simulink model "c_spacecraft_control_sensors_noise_removal"  (R2022a)
settings: Solver=ode45  StartTime=0.0  StopTime=30  RelTol=1e-3
undefined symbols (not defined in the file): Continuous, Time
libraries: slpidlib x3, aerolibnav x1, ctrlSharedLib x1, simulink x1, robotcorelib x1
settings Model: Creator=HP  LastModifiedBy=HP

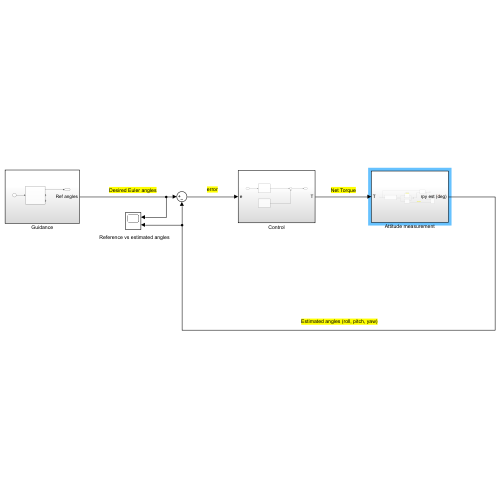
[thumbnail: Simulink's stored preview of the top-level diagram]
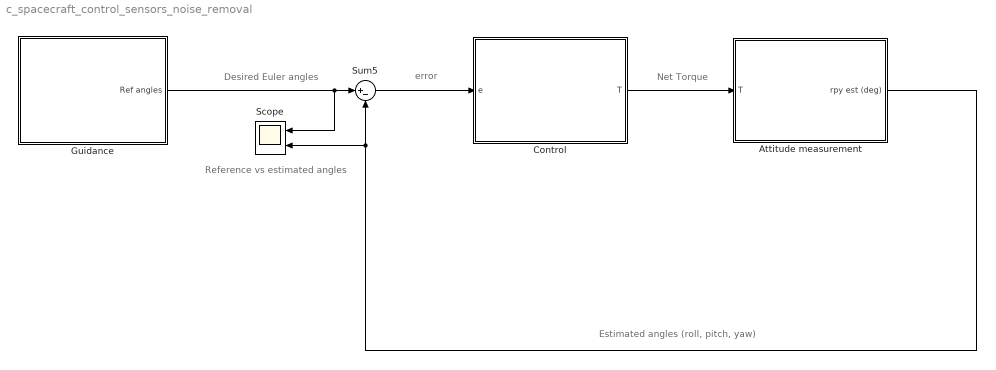
== system c_spacecraft_control_sensors_noise_removal ==
  note: Reference vs estimated angles
  note: Desired Euler angles
  note: Net Torque
  note: error
  note: Estimated angles (roll, pitch, yaw)
  Attitude measurement : Subsystem
  Control : Subsystem
  Guidance : Subsystem
  Scope : Scope  NumInputPorts=2
  Sum5 : Sum  Inputs=|+-
  wires:
  Guidance/1(Ref angles) -> Scope/1, Sum5/1
  Sum5/1 -> Control/1(e)
  Control/1(T) -> Attitude measurement/1(T)
  Attitude measurement/1(rpy est (deg)) -> Sum5/2, Scope/2

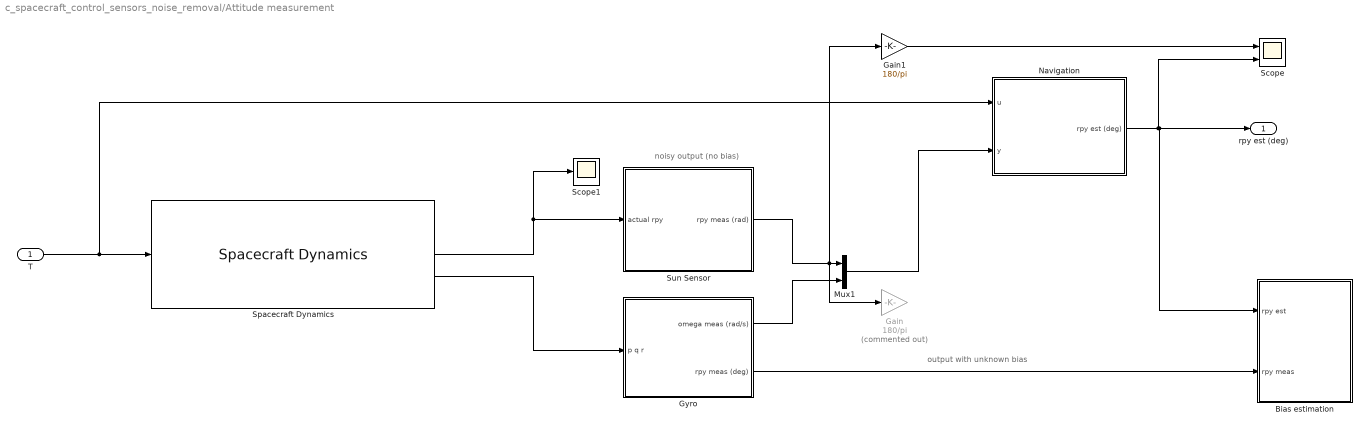
== system c_spacecraft_control_sensors_noise_removal/Attitude measurement ==
  note: noisy output (no bias)
  note: output with unknown bias
  T : Inport
  Bias estimation : Subsystem
  Gain : Gain  Commented=on  Gain=180/pi
  Gain1 : Gain  Gain=180/pi
  Gyro : Subsystem
  Mux1 : Mux  Inputs=2
  Navigation : Subsystem
  Scope : Scope  NumInputPorts=2
  Scope1 : Scope
  Spacecraft Dynamics : SpacecraftDynamics  forcesIn=off  dateOut=off  mass=1000.0  inertia=[2500, 0, 0; 0, 2300, 0; 0, 0, 3000]  orbitType=Circular equatorial  semiMajorAxis=7078000  attitudeFormat=Euler angles  attitude=[10 10 10]  rotationOrder=XYZ  useGravGrad=off  outputTransform=on
  Sun Sensor : Subsystem
  rpy est (deg) : Outport
  wires:
  T/1 -> Spacecraft Dynamics/1, Navigation/1(u)
  Spacecraft Dynamics/3 -> Scope1/1, Sun Sensor/1(actual rpy)
  Spacecraft Dynamics/4 -> Gyro/1(p q r)
  Sun Sensor/1(rpy meas (rad)) -> Gain/1, Mux1/1, Gain1/1
  Gyro/1(omega meas (rad/s)) -> Mux1/2
  Gyro/2(rpy meas (deg)) -> Bias estimation/2(rpy meas)
  Mux1/1 -> Navigation/2(y)
  Navigation/1(rpy est (deg)) -> Bias estimation/1(rpy est), rpy est (deg)/1, Scope/2
  Gain1/1 -> Scope/1

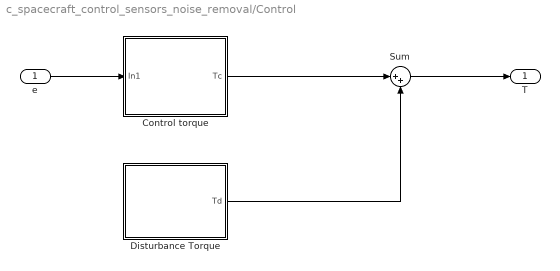
== system c_spacecraft_control_sensors_noise_removal/Control ==
  e : Inport
  Control torque : Subsystem
  Disturbance Torque : Subsystem
  Sum : Sum  Inputs=|++
  T : Outport
  wires:
  e/1 -> Control torque/1(In1)
  Sum/1 -> T/1
  Control torque/1(Tc) -> Sum/1
  Disturbance Torque/1(Td) -> Sum/2

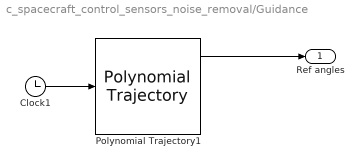
== system c_spacecraft_control_sensors_noise_removal/Guidance ==
  Clock1 : Clock
  Polynomial Trajectory1 : robotcorelib/Polynomial Trajectory  WaypointSource=Internal  Waypoints=[0, 0, 0, 0, 0; 0, 0, 0, 0, 0; 0, 0, 0, 0, 0]  TimePoints=[0,1,2,3,4]  TimeInterval=[ 1, 4 ]  Method=Cubic Polynomial  ParameterSource=Internal  VelocityBoundaryCondition=zeros( 3, 5 )  AccelerationBoundaryCondition=zeros( 2, 5 )  SimulateUsing=Interpreted execution
      settings: SourceProductBaseCode=RO,NV,RR,UV
  Ref angles : Outport
  wires:
  Clock1/1 -> Polynomial Trajectory1/1
  Polynomial Trajectory1/1 -> Ref angles/1

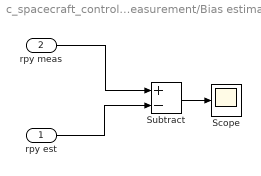
== system c_spacecraft_control_sensors_noise_removal/Attitude measurement/Bias estimation ==
  rpy est : Inport
  rpy meas : Inport  Port=2
  Scope : Scope
  Subtract : Sum  Inputs=+-
  wires:
  Subtract/1 -> Scope/1
  rpy meas/1 -> Subtract/1
  rpy est/1 -> Subtract/2

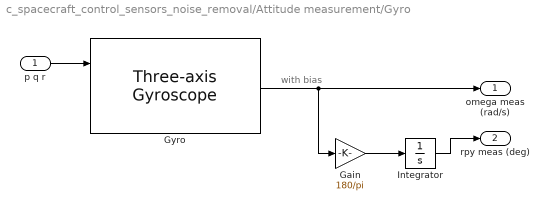
== system c_spacecraft_control_sensors_noise_removal/Attitude measurement/Gyro ==
  note: with bias
  p q r : Inport
  Gain : Gain  Gain=180/pi
  Gyro : aerolibnav/Three-axis Gyroscope  dtype_g=on  w_g=190  z_g=0.707  g_sf_cc=[1 0 0; 0 1 0; 0 0 1]  g_bias=[0.1 -0.1 0.15]  g_sen=[0 0 0]  g_Ts=0  g_rand=off  g_seeds=[1 1 1]  g_pow=[0.1 0.1 0.1]  g_sat="[-inf  -inf  -inf  inf inf inf]"
      settings: SourceProductBaseCode=AE
  Integrator : Integrator  InitialCondition=10
  omega meas (rad/s) : Outport
  rpy meas (deg) : Outport  Port=2
  wires:
  p q r/1 -> Gyro/1
  Gyro/1 -> omega meas (rad/s)/1, Gain/1
  Integrator/1 -> rpy meas (deg)/1
  Gain/1 -> Integrator/1

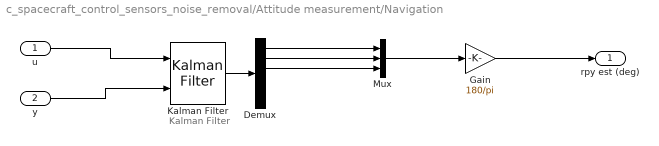
== system c_spacecraft_control_sensors_noise_removal/Attitude measurement/Navigation ==
  note: Kalman Filter
  u : Inport
  y : Inport  Port=2
  Demux : Demux  Outputs=6
  Gain : Gain  Gain=180/pi
  Kalman Filter : ctrlSharedLib/Kalman Filter  TimeDomain=Continuous-Time  UseCurrentEstimator=on  ModelSource=Individual A, B, C, D matrices  ModelSourceVariable=ss(0.95,1,1,0,1)  A=[0 0 0 1 0 0; 0 0 0 0 1 0; 0 0 0 0 0 1; 9.44e-7 0 0 0 0 0;0 7.33e-5 0 0 0 0;0 0 0 -7.1e-5 0 0]  B=[0 0 0;0 0 0;0 0 0;4e-4 0 0;0 4.35e-4 0; 0 0 3.33e-4]  C=[1 0 0 0 0 0;0 1 0 0 0 0;0 0 1 0 0 0;0 0 0 1 0 0;0 0 0 0 1 0;0 0 0 0 0 1]  D=0  NumberOfStates=1  NumberOfInputs=1  NumberOfOutputs=1  InitialEstimateSource=Dialog  X0=[0.174 0.174 0.174 0 0 0]  P0=10  UseK=off  UseGH=off  NumberOfProcessNoiseInputs=1  G=1  TimeInvariantG=on  H=0  TimeInvariantH=on  Q=0.01  TimeInvariantQ=on  R=1  TimeInvariantR=on  N=0  TimeInvariantN=on  AddInputPort=on  AddEnablePort=off  OutputEstimatedY=off  OutputP=off  Ts=-1
  Mux : Mux  Inputs=3
  rpy est (deg) : Outport
  wires:
  Demux/1 -> Mux/1
  Demux/2 -> Mux/2
  Mux/1 -> Gain/1
  Demux/3 -> Mux/3
  Kalman Filter/1 -> Demux/1
  Gain/1 -> rpy est (deg)/1
  u/1 -> Kalman Filter/1
  y/1 -> Kalman Filter/2

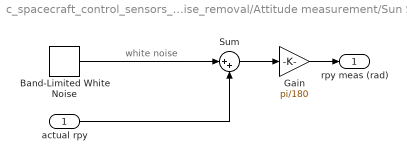
== system c_spacecraft_control_sensors_noise_removal/Attitude measurement/Sun Sensor ==
  note: white noise
  actual rpy : Inport
  Band-Limited White Noise : simulink/Sources/Band-Limited White Noise  Cov=[0.1 0.1 0.1]  Ts=0.1  seed=[23341]
  Gain : Gain  Gain=pi/180
  Sum : Sum  Inputs=|++
  rpy meas (rad) : Outport
  wires:
  Band-Limited White Noise/1 -> Sum/1
  actual rpy/1 -> Sum/2
  Sum/1 -> Gain/1
  Gain/1 -> rpy meas (rad)/1

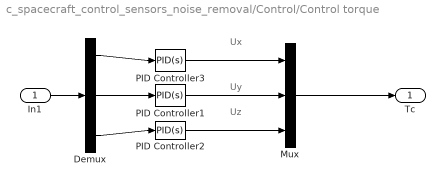
== system c_spacecraft_control_sensors_noise_removal/Control/Control torque ==
  note: Uz
  note: Uy
  note: Ux
  In1 : Inport
  Demux : Demux  Outputs=3
  Mux : Mux  Inputs=3
  PID Controller1 : slpidlib/PID Controller  Controller=PID  Form=Parallel  TimeDomain=Continuous-time  UseExternalTs=off  SampleTime=-1  IntegratorMethod=Forward Euler  FilterMethod=Forward Euler  ControllerParametersSource=internal  P=185.063851638376  I=45.953859056055  UseKiTs=off  D=181.02375970947  N=47.9472510450487  UseFilter=on  TunerSelectOption=Transfer Function Based (PID Tuner App)  InitialConditionSource=internal  InitialConditionForIntegrator=0  InitialConditionForFilter=0  DifferentiatorICPrevScaledInput=0  ExternalReset=none  TrackingMode=off  Kt=1  LimitOutput=off  SatLimitsSource=internal  UpperSaturationLimit=inf  LowerSaturationLimit=-inf  LinearizeAsGain=on  AntiWindupMode=none  Kb=1  POutMin=[]  POutMax=[]  IOutMin=[]  IOutMax=[]  DOutMin=[]  DOutMax=[]  NOutMin=[]  NOutMax=[]  SumOutMin=[]  SumOutMax=[]  SaturationOutMin=[]  SaturationOutMax=[]  PParamMin=[]  PParamMax=[]  IParamMin=[]  IParamMax=[]  DParamMin=[]  DParamMax=[]  NParamMin=[]  NParamMax=[]  KbParamMin=[]  KbParamMax=[]  KtParamMin=[]  KtParamMax=[]  KbOutMin=[]  KbOutMax=[]  KtOutMin=[]  KtOutMax=[]  IntegratorOutMin=[]  IntegratorOutMax=[]  FilterOutMin=[]  FilterOutMax=[]  SumI1OutMin=[]  SumI1OutMax=[]  SumI2OutMin=[]  SumI2OutMax=[]  SumI3OutMin=[]  SumI3OutMax=[]  SumI4OutMin=[]  SumI4OutMax=[]  SumDOutMin=[]  SumDOutMax=[]  DifferentiatorOutMin=[]  DifferentiatorOutMax=[]  FilterDiffOutCoefMin=[]  FilterDiffOutCoefMax=[]  ReciprocalOutMin=[]  ReciprocalOutMax=[]  SumDenOutMin=[]  SumDenOutMax=[]  SumNumOutMin=[]  SumNumOutMax=[]  DivideOutMin=[]  DivideOutMax=[]  UdiffTsProdOutMin=[]  UdiffTsProdOutMax=[]  NTsProdOutMin=[]  NTsProdOutMax=[]  UintegralTsProdOutMin=[]  UintegralTsProdOutMax=[]  UngainTsProdOutMin=[]  UngainTsProdOutMax=[]  IntegratorContinuousStateAttributes=''  IntegratorStateMustResolveToSignalObject=off  IntegratorRTWStateStorageClass=Auto  FilterContinuousStateAttributes=''  FilterStateMustResolveToSignalObject=off  FilterRTWStateStorageClass=Auto  ParallelPVariant=InternalParameters  IdealPVariant=Disabled  IVariant=InternalParameters  DVariant=InternalParameters  IntegratorVariant=Continuous  SatVariant=Disabled  AWVariant=Passthrough  PCopyVariant=Disabled  TRVariant=Disabled  FdbkBlocksVariant=Forward  IdealPFdbkVariant=Disabled  SatFdbkVariant=Disabled  DerivativeFilterVariant=ContFilter  NVariant=InternalParameters  NCopyVariant=Disabled  FilterICVariant=InternalICsFilter  IntegratorICVariant=InternalICs  ExternalResetVariant=Disabled  TRSumVariant=Passthrough  SumFdbkVariant=Disabled  SumVariant=Sum_PID  TsampFilterVariant=InternalTs  TsampNgainVariant=Passthrough  TsampIntegralVariant=Passthrough  ExternalSaturationOutDataTypeStr=Inherit: Same as second input  aMode=0
  PID Controller2 : slpidlib/PID Controller  Controller=PID  Form=Parallel  TimeDomain=Continuous-time  UseExternalTs=off  SampleTime=-1  IntegratorMethod=Forward Euler  FilterMethod=Forward Euler  ControllerParametersSource=internal  P=65  I=15  UseKiTs=off  D=85  N=5.45397025421619  UseFilter=on  TunerSelectOption=Transfer Function Based (PID Tuner App)  InitialConditionSource=internal  InitialConditionForIntegrator=0  InitialConditionForFilter=0  DifferentiatorICPrevScaledInput=0  ExternalReset=none  TrackingMode=off  Kt=1  LimitOutput=off  SatLimitsSource=internal  UpperSaturationLimit=inf  LowerSaturationLimit=-inf  LinearizeAsGain=on  AntiWindupMode=none  Kb=1  POutMin=[]  POutMax=[]  IOutMin=[]  IOutMax=[]  DOutMin=[]  DOutMax=[]  NOutMin=[]  NOutMax=[]  SumOutMin=[]  SumOutMax=[]  SaturationOutMin=[]  SaturationOutMax=[]  PParamMin=[]  PParamMax=[]  IParamMin=[]  IParamMax=[]  DParamMin=[]  DParamMax=[]  NParamMin=[]  NParamMax=[]  KbParamMin=[]  KbParamMax=[]  KtParamMin=[]  KtParamMax=[]  KbOutMin=[]  KbOutMax=[]  KtOutMin=[]  KtOutMax=[]  IntegratorOutMin=[]  IntegratorOutMax=[]  FilterOutMin=[]  FilterOutMax=[]  SumI1OutMin=[]  SumI1OutMax=[]  SumI2OutMin=[]  SumI2OutMax=[]  SumI3OutMin=[]  SumI3OutMax=[]  SumI4OutMin=[]  SumI4OutMax=[]  SumDOutMin=[]  SumDOutMax=[]  DifferentiatorOutMin=[]  DifferentiatorOutMax=[]  FilterDiffOutCoefMin=[]  FilterDiffOutCoefMax=[]  ReciprocalOutMin=[]  ReciprocalOutMax=[]  SumDenOutMin=[]  SumDenOutMax=[]  SumNumOutMin=[]  SumNumOutMax=[]  DivideOutMin=[]  DivideOutMax=[]  UdiffTsProdOutMin=[]  UdiffTsProdOutMax=[]  NTsProdOutMin=[]  NTsProdOutMax=[]  UintegralTsProdOutMin=[]  UintegralTsProdOutMax=[]  UngainTsProdOutMin=[]  UngainTsProdOutMax=[]  IntegratorContinuousStateAttributes=''  IntegratorStateMustResolveToSignalObject=off  IntegratorRTWStateStorageClass=Auto  FilterContinuousStateAttributes=''  FilterStateMustResolveToSignalObject=off  FilterRTWStateStorageClass=Auto  ParallelPVariant=InternalParameters  IdealPVariant=Disabled  IVariant=InternalParameters  DVariant=InternalParameters  IntegratorVariant=Continuous  SatVariant=Disabled  AWVariant=Passthrough  PCopyVariant=Disabled  TRVariant=Disabled  FdbkBlocksVariant=Forward  IdealPFdbkVariant=Disabled  SatFdbkVariant=Disabled  DerivativeFilterVariant=ContFilter  NVariant=InternalParameters  NCopyVariant=Disabled  FilterICVariant=InternalICsFilter  IntegratorICVariant=InternalICs  ExternalResetVariant=Disabled  TRSumVariant=Passthrough  SumFdbkVariant=Disabled  SumVariant=Sum_PID  TsampFilterVariant=InternalTs  TsampNgainVariant=Passthrough  TsampIntegralVariant=Passthrough  ExternalSaturationOutDataTypeStr=Inherit: Same as second input  aMode=0
  PID Controller3 : slpidlib/PID Controller  Controller=PID  Form=Parallel  TimeDomain=Continuous-time  UseExternalTs=off  SampleTime=-1  IntegratorMethod=Forward Euler  FilterMethod=Forward Euler  ControllerParametersSource=internal  P=185.063851638376  I=45.953859056055  UseKiTs=off  D=181.02375970947  N=47.9472510450487  UseFilter=on  TunerSelectOption=Transfer Function Based (PID Tuner App)  InitialConditionSource=internal  InitialConditionForIntegrator=0  InitialConditionForFilter=0  DifferentiatorICPrevScaledInput=0  ExternalReset=none  TrackingMode=off  Kt=1  LimitOutput=off  SatLimitsSource=internal  UpperSaturationLimit=inf  LowerSaturationLimit=-inf  LinearizeAsGain=on  AntiWindupMode=none  Kb=1  POutMin=[]  POutMax=[]  IOutMin=[]  IOutMax=[]  DOutMin=[]  DOutMax=[]  NOutMin=[]  NOutMax=[]  SumOutMin=[]  SumOutMax=[]  SaturationOutMin=[]  SaturationOutMax=[]  PParamMin=[]  PParamMax=[]  IParamMin=[]  IParamMax=[]  DParamMin=[]  DParamMax=[]  NParamMin=[]  NParamMax=[]  KbParamMin=[]  KbParamMax=[]  KtParamMin=[]  KtParamMax=[]  KbOutMin=[]  KbOutMax=[]  KtOutMin=[]  KtOutMax=[]  IntegratorOutMin=[]  IntegratorOutMax=[]  FilterOutMin=[]  FilterOutMax=[]  SumI1OutMin=[]  SumI1OutMax=[]  SumI2OutMin=[]  SumI2OutMax=[]  SumI3OutMin=[]  SumI3OutMax=[]  SumI4OutMin=[]  SumI4OutMax=[]  SumDOutMin=[]  SumDOutMax=[]  DifferentiatorOutMin=[]  DifferentiatorOutMax=[]  FilterDiffOutCoefMin=[]  FilterDiffOutCoefMax=[]  ReciprocalOutMin=[]  ReciprocalOutMax=[]  SumDenOutMin=[]  SumDenOutMax=[]  SumNumOutMin=[]  SumNumOutMax=[]  DivideOutMin=[]  DivideOutMax=[]  UdiffTsProdOutMin=[]  UdiffTsProdOutMax=[]  NTsProdOutMin=[]  NTsProdOutMax=[]  UintegralTsProdOutMin=[]  UintegralTsProdOutMax=[]  UngainTsProdOutMin=[]  UngainTsProdOutMax=[]  IntegratorContinuousStateAttributes=''  IntegratorStateMustResolveToSignalObject=off  IntegratorRTWStateStorageClass=Auto  FilterContinuousStateAttributes=''  FilterStateMustResolveToSignalObject=off  FilterRTWStateStorageClass=Auto  ParallelPVariant=InternalParameters  IdealPVariant=Disabled  IVariant=InternalParameters  DVariant=InternalParameters  IntegratorVariant=Continuous  SatVariant=Disabled  AWVariant=Passthrough  PCopyVariant=Disabled  TRVariant=Disabled  FdbkBlocksVariant=Forward  IdealPFdbkVariant=Disabled  SatFdbkVariant=Disabled  DerivativeFilterVariant=ContFilter  NVariant=InternalParameters  NCopyVariant=Disabled  FilterICVariant=InternalICsFilter  IntegratorICVariant=InternalICs  ExternalResetVariant=Disabled  TRSumVariant=Passthrough  SumFdbkVariant=Disabled  SumVariant=Sum_PID  TsampFilterVariant=InternalTs  TsampNgainVariant=Passthrough  TsampIntegralVariant=Passthrough  ExternalSaturationOutDataTypeStr=Inherit: Same as second input  aMode=0
  Tc : Outport
  wires:
  Mux/1 -> Tc/1
  In1/1 -> Demux/1
  Demux/1 -> PID Controller3/1
  Demux/2 -> PID Controller1/1
  Demux/3 -> PID Controller2/1
  PID Controller3/1 -> Mux/1
  PID Controller1/1 -> Mux/2
  PID Controller2/1 -> Mux/3

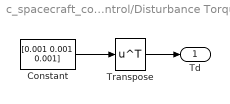
== system c_spacecraft_control_sensors_noise_removal/Control/Disturbance Torque ==
  Constant : Constant  Value=[0.001 0.001 0.001]  VectorParams1D=off
  Transpose : Math  Operator=transpose
  Td : Outport
  wires:
  Transpose/1 -> Td/1
  Constant/1 -> Transpose/1
